simulink model "trajectory_generator_sim"  (R2022a)
settings: Solver=FixedStepAuto  StartTime=0.0  StopTime=8  FixedStep=0.0001  RelTol=1e-3
values from neighbouring files (symbols this model uses):
  Acc_data = Calculate_Acceleration_instants(H(ii,:),H(ii+1,:),v_max,a_max)    [Stitch_trajectory.m]    (also in func_Stitch_trajectory.m = func_Calculate_Acceleration_instants(H(ii,:),H(ii+1,:),v_max; simulink_runner.m = Calculate_Acceleration_instants(Rc,Rd,v_max,a_max))
settings Model: Creator=Ankit  LastModifiedBy=Ankit

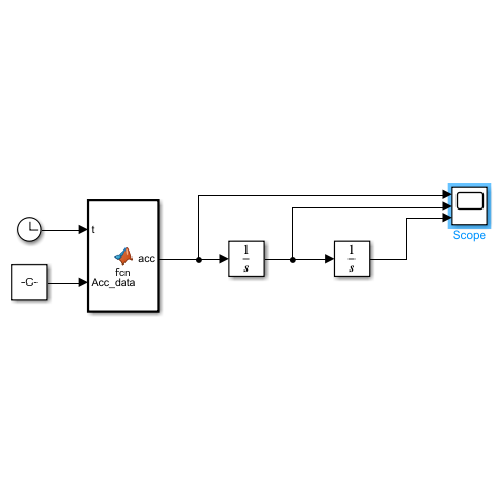
[thumbnail: Simulink's stored preview of the top-level diagram]
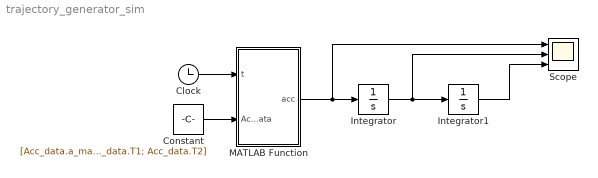
== system trajectory_generator_sim ==
  Clock : Clock
  Constant : Constant  Value=[Acc_data.a_max; Acc_data.T1; Acc_data.T2]
  Integrator : Integrator
  Integrator1 : Integrator
  MATLAB Function : MATLAB Function  TreatAsAtomicUnit=on
  Scope : Scope  NumInputPorts=3
  wires:
  Clock/1 -> MATLAB Function/1(t)
  MATLAB Function/1(acc) -> Scope/1, Integrator/1
  Constant/1 -> MATLAB Function/2(Acc_data)
  Integrator1/1 -> Scope/3
  Integrator/1 -> Scope/2, Integrator1/1

== matlab function trajectory_generator_sim/MATLAB Function ==
  data: t input; acc output; Acc_data input
function acc = fcn(t,Acc_data)

a_max = Acc_data(1);
T1 = Acc_data(2);
T2 = Acc_data(3);
Tf = T1+T2;
acc = a_max;
if t>=T1 && t < T2
    acc = 0;
elseif t >= T2 && t < Tf
    acc = -a_max;
elseif t >= Tf 
    acc = 0;
end
